simulink model "chopper"  (Simulink 8.8)
settings: Solver=ode23tb  StartTime=0.0  StopTime=10  RelTol=1e-4
InitFcn:
  | load power_dcdrive_init
libraries: powerlib x25
Description:
  | The 'Model  initialization function' defined in the
  | 
  | Model Properties loads the  initial states vector
  | 
  | 'xInitial' saved in the power_dcdrive_init.mat file.
  | 
  | 
  | 
  | To start in steady state with Speed = 120 rad/s
  | 
  | and Torque = 5 N.m/s, check 'Initial state' in
  | 
  | Simulation/Simulation parameters/Workspace I/O.
  | 
  | 
  | Copyright 2008 The MathWorks(TM), Inc.
settings Model: SuppressorTable=22 serialization::archive 11 0 3 0 0 0 0 0  Creator=Hoand Lehuy, Laval University  LastModifiedBy=sithuaung  ExtModeTrigMode=oneshot  ExtModeArmWhenConnect=off  ExtModeAutoUpdateStatusClock=off
settings DataIOCC: LimitDataPoints=off  SaveOutput=off  SignalLogging=off  SaveTime=off  SignalLoggingName=sigsOut
settings OptimizationCC: BlockReduction=off  BooleanDataType=off  ExpressionDepthLimit=2147483647  InitFltsAndDblsToZero=on  EfficientMapNaN2IntZero=off
settings DebuggingCC: SaveWithParameterizedLinksMsg=none  CheckExecutionContextPreStartOutputMsg=on  CheckExecutionContextRuntimeOutputMsg=on  SignalResolutionControl=TryResolveAllWithWarning  MultiTaskDSMMsg=warning  MultiTaskCondExecSysMsg=none  UnconnectedInputMsg=none  UnconnectedOutputMsg=none  StrictBusMsg=None
settings HardwareCC: TargetUnknown=on
settings GRTTargetCC: TargetFcnLib=ansi_tfl_tmw.mat

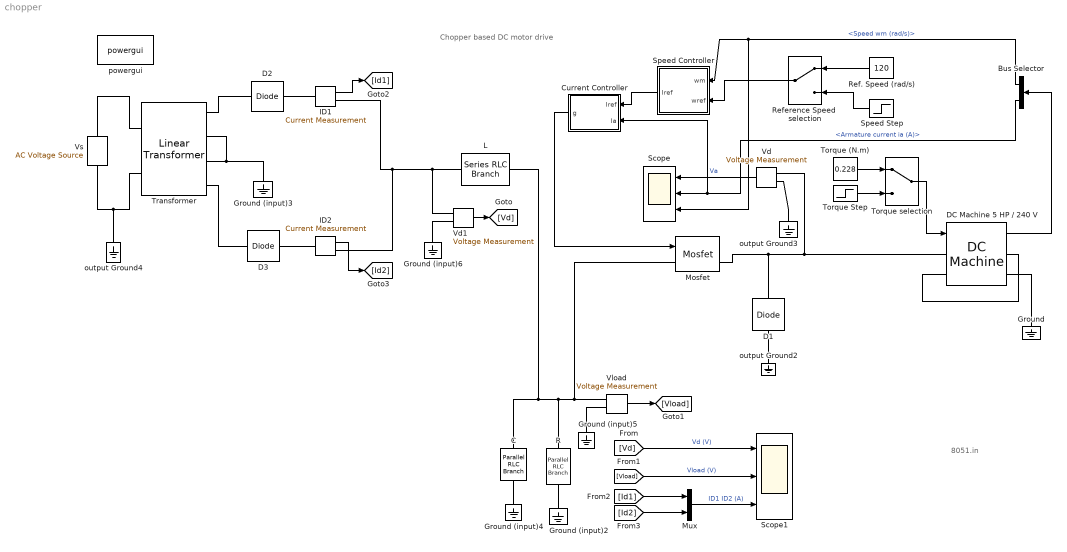
== system chopper ==
  note: Chopper based DC motor drive
  note: 8051.in
  Bus Selector : BusSelector  OutputSignals=Speed wm (rad/s),Armature current ia (A)
  C : powerlib/Elements/Parallel RLC Branch  LConnTagsString=a  RConnTagsString=__new0  BranchType=C  Resistance=5  Inductance=1.0  SetiL0=off  InitialCurrent=0  Capacitance=500e-06  Setx0=off  InitialVoltage=0  Measurements=None
  Current Controller : Subsystem  mask{h=1}
      mask prompts: h "Hysteresis band (A)"
      mask help: Hysteresis Current Controller
      mask Display: plot(0,0,100,100,[45,45],[35,65],[55,55],[35,65],[45,65],[65,65],[35,55],[35,35])
  D1 : powerlib/Power Electronics/Diode  Ron=0.05  Lon=0  Vf=0.7  IC=0  UseSnubber=off  Rs=Inf  Cs=0.1e-6  Measurements=off
  D2 : powerlib/Power Electronics/Diode  Ron=1e-3  Lon=0  Vf=0.7  IC=0  UseSnubber=off  Rs=1e6  Cs=inf  Measurements=off
  D3 : powerlib/Power Electronics/Diode  Ron=1e-3  Lon=0  Vf=0.7  IC=0  UseSnubber=off  Rs=1e6  Cs=inf  Measurements=off
  DC Machine 5 HP / 240 V : powerlib/Machines/DC Machine  PresetModel=No  MechanicalLoad=Torque TL  FieldType=Wound  ShowDetailedParameters=on  MeasurementBus=off  RLa="[ 7.061  0.058]"  RLf="[ 12.939  0.531]"  Laf=0.0662  MachineConstant=Torque constant (N.m/A)  Ke=1.8  Kt=1.8  J=0.21e-3  Bm=0  Tf=0  w0=1  Ifinit=-8.465390e-22  TsPowergui=0  TsBlock=-1
  Ground : powerlib/Elements/Ground  LConnTagsString=a
  Ground (input){2..6} (5 alike) : powerlib/Elements/Ground  LConnTagsString=a
  ID1 : powerlib/Measurements/Current Measurement  PhasorSimulation=off  OutputType=Complex  PSBequivalent=0
  ID2 : powerlib/Measurements/Current Measurement  PhasorSimulation=off  OutputType=Complex  PSBequivalent=0
  L : powerlib/Elements/Series RLC Branch  LConnTagsString=__new0  RConnTagsString=__new0  BranchType=L  Resistance=1.0  Inductance=20e-03  SetiL0=off  InitialCurrent=0  Capacitance=1.0  Setx0=off  InitialVoltage=0  Measurements=None
  Mosfet : powerlib/Power Electronics/Mosfet  Ron=0.1  Lon=0  Rd=0.01  Vfd=0  IC=0  Rs=1e5  Cs=inf  Measurements=on
  Mux : Mux  Inputs=2
  R : powerlib/Elements/Parallel RLC Branch  LConnTagsString=a  RConnTagsString=__new0  BranchType=R  Resistance=10  Inductance=1.0  SetiL0=off  InitialCurrent=0  Capacitance=200e-06  Setx0=off  InitialVoltage=0  Measurements=None
  Ref. Speed (rad/s) : Constant  Value=120
  Reference Speed  selection : ManualSwitch
  Scope : Scope  NumInputPorts=3
  Scope1 : Scope  NumInputPorts=3
  Speed Controller : Subsystem  mask(PI controller){Kp=0.9, Ki=0.01, Ilim=4}
      mask prompts: Kp "Proportional gain (Kp)"; Ki "Integral gain (Ki)"; Ilim "Current limit (A)"
      mask help: Proportional-Integral Speed Controller
      mask Display: plot(0,0,100,100,[35,35,65],[70,30,30],[35,65],[45,60])
  Speed Step : Step  Time=0.4  Before=120  After=160  SampleTime=0
  Torque selection : ManualSwitch
  Torque (N.m) : Constant  Value=0.228
  Torque Step : Step  Time=1.2  Before=5  After=25  SampleTime=0
  Transformer : powerlib/Elements/Linear Transformer  UNITS=SI  NominalPower=[50 50]  winding1=[250 0 0]  winding2=[230 0 0.01]  ThreeWindings=on  winding3=[230 0 0.01]  RmLm=[Inf Inf]  Measurements=None  DataType=on
  Vd : powerlib/Measurements/Voltage Measurement  Tag=PoWeRsYsTeMmEaSuReMeNt  PhasorSimulation=off  OutputType=Magnitude  PSBequivalent=0
  Vd1 : powerlib/Measurements/Voltage Measurement  Tag=PoWeRsYsTeMmEaSuReMeNt  PhasorSimulation=off  OutputType=Magnitude  PSBequivalent=0
  Vload : powerlib/Measurements/Voltage Measurement  Tag=PoWeRsYsTeMmEaSuReMeNt  PhasorSimulation=off  OutputType=Magnitude  PSBequivalent=0
  Vs : powerlib/Electrical Sources/AC Voltage Source  Description=source block  Amplitude=400  Phase=0  Frequency=50  SampleTime=0  Measurements=None  BusType=swing  Pref=10e3  Qref=0  Qmin=-inf  Qmax=+inf
      settings: AttributesFormatString=\n
  output Ground2 : powerlib/Elements/Ground  LConnTagsString=a
  output Ground3 : powerlib/Elements/Ground  LConnTagsString=a
  output Ground4 : powerlib/Elements/Ground  LConnTagsString=a
  powergui : powerlib/powergui  SimulationMode=Continuous  SolverType=Tustin/Backward Euler (TBE)  SampleTime=0  frequency=60  SPID=off  DisableSnubberDevices=off  DisableRonSwitches=off  DisableVfSwitches=off  SwTol=0  DisplayEquations=off  Interpol=off  ExternalGateDelay=off  methode=off  Ts=0  FunctionMessages=off  echomessages=off  HookPort=off  EnableUseOfTLC=off  x0status=blocks  frequencyindice=0  Pbase=100e6  ErrMax=1e-4  Iterations=50  UnitsV=kV  UnitsW=MW  buscounter=0  RestoreLinks=warning  ResistiveCurrentMeasurement=off  Frange=[0:2:500]  Ylog=off  Xlog=on  ShowGrid=off  save=off  variable=ZData  structure=ScopeData  ZoomFFT=off  StartTime=0.0  cycles=1  DisplayStyle=1  fundamental=60  FreqAxis=off  MaxFrequency=1000  frequencyindicesteady=1  RmsSteady=1  display=off
  wires:
  Speed Controller/1(Iref) -> Current Controller/1(Iref)
  Bus Selector/1 -> Speed Controller/1(wm), Scope/3  "<Speed wm (rad/s)>"
  Bus Selector/2 -> Scope/2, Current Controller/2(Ia)  "<Armature current ia (A)>"
  Current Controller/1(g) -> Mosfet/1
  Vd/1 -> Scope/1  "Va"
  DC Machine 5 HP / 240 V/1 -> Bus Selector/1
  Torque (N.m)/1 -> Torque selection/1
  Torque Step/1 -> Torque selection/2
  Torque selection/1 -> DC Machine 5 HP / 240 V/1
  Ref. Speed (rad/s)/1 -> Reference Speed  selection/1
  Speed Step/1 -> Reference Speed  selection/2
  Reference Speed  selection/1 -> Speed Controller/2(wref)
  Vd1/1 -> [Vd]
  Vload/1 -> [Vload]
  ID1/1 -> [Id1]
  ID2/1 -> [Id2]
  [Vd] -> Scope1/1  "Vd (V)"
  [Vload] -> Scope1/2  "Vload (V)"
  Mux/1 -> Scope1/3  "ID1 ID2 (A)"
  [Id1] -> Mux/1
  [Id2] -> Mux/2
  connections:
  output Ground2/LConn1 -- D1/LConn1
  Mosfet/RConn1 -- DC Machine 5 HP / 240 V/LConn1 -- Vd/LConn1 -- D1/RConn1
  output Ground3/LConn1 -- Vd/LConn2
  DC Machine 5 HP / 240 V/LConn2 -- DC Machine 5 HP / 240 V/RConn1
  output Ground4/LConn1 -- Transformer/LConn2 -- Vs/LConn1
  Vload/LConn1 -- R/LConn1 -- C/LConn1 -- L/RConn1 -- Mosfet/LConn1
  Ground (input)3/LConn1 -- Transformer/RConn2 -- Transformer/RConn3
  ID2/RConn1 -- L/LConn1 -- Vd1/LConn1 -- ID1/RConn1
  Vs/RConn1 -- Transformer/LConn1
  Transformer/RConn1 -- D2/LConn1
  Transformer/RConn4 -- D3/LConn1
  Ground (input)4/LConn1 -- C/RConn1
  Ground (input)2/LConn1 -- R/RConn1
  Ground (input)5/LConn1 -- Vload/LConn2
  D2/RConn1 -- ID1/LConn1
  D3/RConn1 -- ID2/LConn1
  Vd1/LConn2 -- Ground (input)6/LConn1
  DC Machine 5 HP / 240 V/RConn2 -- Ground/LConn1

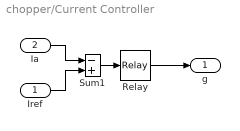
== system chopper/Current Controller ==
  Iref : Inport
  Ia : Inport  Port=2
  Relay : Relay  OnSwitchValue=h/2  OffSwitchValue=-h/2
  Sum1 : Sum  Inputs=-+  SaturateOnIntegerOverflow=on  InputSameDT=on  OutDataTypeStr=Inherit: Same as first input
  g : Outport  InitialOutput=0
  wires:
  Sum1/1 -> Relay/1
  Relay/1 -> g/1
  Ia/1 -> Sum1/1
  Iref/1 -> Sum1/2

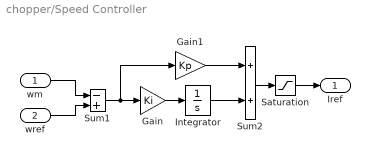
== system chopper/Speed Controller ==
  wm : Inport
  wref : Inport  Port=2
  Gain : Gain  Gain=Ki  SaturateOnIntegerOverflow=on  OutDataTypeStr=Inherit: Same as input  ParamDataTypeStr=Inherit: Same as input
  Gain1 : Gain  Gain=Kp  SaturateOnIntegerOverflow=on  OutDataTypeStr=Inherit: Same as input  ParamDataTypeStr=Inherit: Same as input
  Integrator : Integrator  LimitOutput=on  UpperSaturationLimit=Ilim  LowerSaturationLimit=-Ilim
  Saturation : Saturate  UpperLimit=Ilim  LowerLimit=-Ilim
  Sum1 : Sum  Inputs=-+  SaturateOnIntegerOverflow=on  InputSameDT=on  OutDataTypeStr=Inherit: Same as first input
  Sum2 : Sum  SaturateOnIntegerOverflow=on  InputSameDT=on  OutDataTypeStr=Inherit: Same as first input
  Iref : Outport  InitialOutput=0
  wires:
  Saturation/1 -> Iref/1
  Sum2/1 -> Saturation/1
  Integrator/1 -> Sum2/2
  wref/1 -> Sum1/2
  wm/1 -> Sum1/1
  Sum1/1 -> Gain1/1, Gain/1
  Gain/1 -> Integrator/1
  Gain1/1 -> Sum2/1
